simulink model "testMagnetoField"  (R2021a)
settings: Solver=VariableStepAuto  StartTime=0.0  StopTime=Torb  RelTol=1e-3
settings Model: DataDictionary=databus.sldd  Creator=Laura  LastModifiedBy=Laura

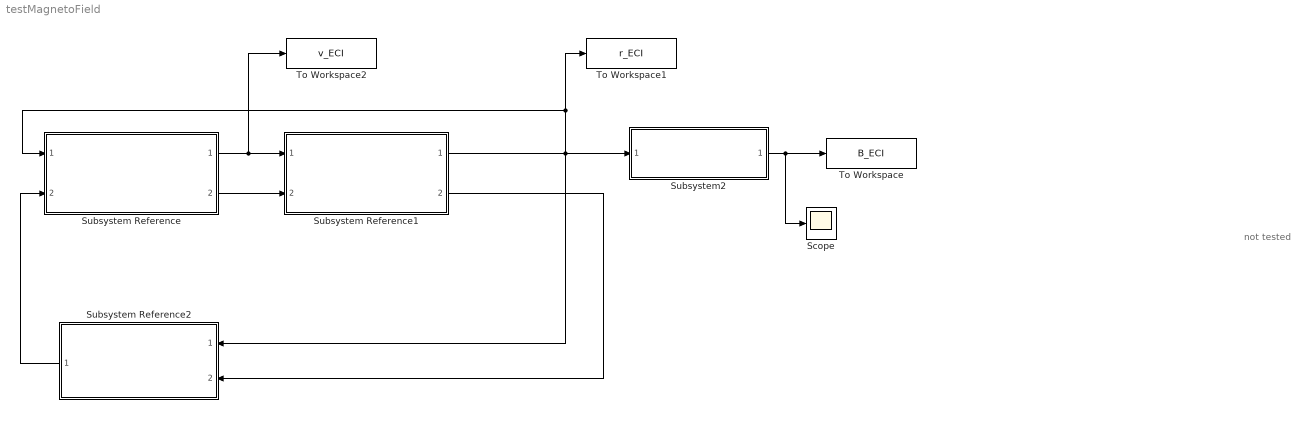
== system testMagnetoField ==
  note: not tested
  Scope : Scope
  Subsystem Reference : Subsystem  ReferencedSubsystem=Dynamics
  Subsystem Reference1 : Subsystem  ReferencedSubsystem=Kinematics
  Subsystem Reference2 : Subsystem  ReferencedSubsystem=GravityTorque
  Subsystem2 : Subsystem  ReferencedSubsystem=MagDipole
  To Workspace : ToWorkspace  VariableName=B_ECI  SaveFormat=Timeseries  SampleTime=-1
  To Workspace1 : ToWorkspace  VariableName=r_ECI  SaveFormat=Timeseries  SampleTime=-1
  To Workspace2 : ToWorkspace  VariableName=v_ECI  SaveFormat=Timeseries  SampleTime=-1
  wires:
  Subsystem Reference2/1 -> Subsystem Reference/2
  Subsystem Reference1/1 -> Subsystem Reference2/1, To Workspace1/1, Subsystem Reference/1, Subsystem2/1
  Subsystem Reference1/2 -> Subsystem Reference2/2
  Subsystem Reference/2 -> Subsystem Reference1/2
  Subsystem Reference/1 -> To Workspace2/1, Subsystem Reference1/1
  Subsystem2/1 -> Scope/1, To Workspace/1
